simulink model "Kalman"  (R2019b)
settings: Solver=VariableStepAuto  StartTime=0.0  StopTime=20  RelTol=1e-3
values from neighbouring files (symbols this model uses):
  A = [0.01   -0.4940 ; 0.1129 -0.3832]    [Initialization.m]
  B = [0.5919 ; 0.5191]    [Initialization.m]
  C = [1 0]    [Initialization.m]
  mn = 0.07    [Initialization.m]
  pn = 0.09    [Initialization.m]
  Ts = -1    [Initialization.m]
undefined symbols (not defined in the file or in its folder): Continuous, sigbuilder_block, Time
libraries: ctrlSharedLib x1
settings Model: Creator=Devan  LastModifiedBy=Devan

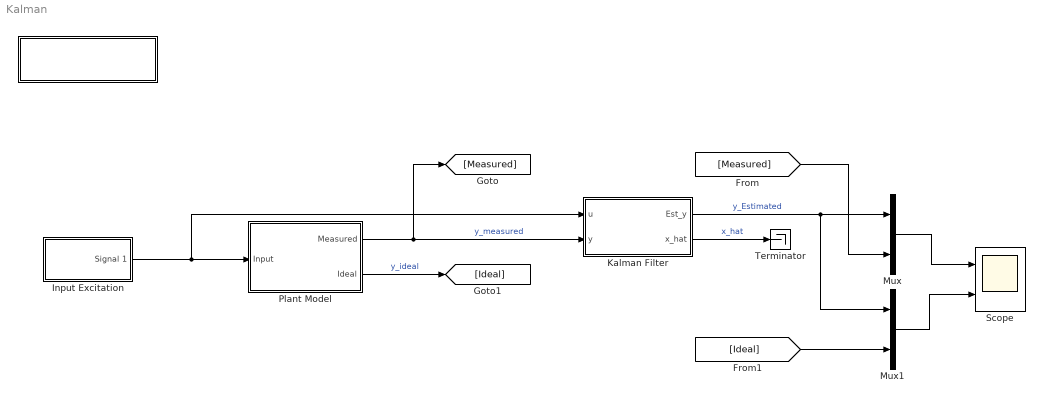
== system Kalman ==
  " " : Subsystem  LoadFcn=run('Initialization.m')  InitFcn=run('Initialization.m')
      settings: OpenFcn=run('Initialization.m')
      mask DialogControl Control3 Prompt: Click to Initialize System
      mask Display: disp('Click to Initialize System')
  Input Excitation : Subsystem  Tag=STV Subsys  LoadFcn=sigbuilder_block('load');  StartFcn=sigbuilder_block('start');  StopFcn=sigbuilder_block('stop');  ClipboardFcn=sigbuilder_block('clipboard');  mask(Sigbuilder block){tuvar=[0:10]}
      mask help: Simulink:masks:SigbuilderBlock_MD
      mask init:
      | if ~strcmp(get_param(bdroot(gcbh),'SimulationStatus'),'stopped') tuvar = sigbuilder_block('maskInit'); end
      settings: CopyFcn=sigbuilder_block('copy');  DeleteFcn=sigbuilder_block('delete');  ModelCloseFcn=sigbuilder_block('modelClose');  PreSaveFcn=sigbuilder_block('preSave');  PauseFcn=sigbuilder_block('pause');  ContinueFcn=sigbuilder_block('continue');  NameChangeFcn=sigbuilder_block('namechange');  OpenFcn=sigbuilder_block('open',[211.5 97.5 550.5 362.5 ]);  CloseFcn=sigbuilder_block('close');
      mask Display: plot(0, 0, 100, 100,[2, 2, 32, 32, 2], [68, 8, 8, 68, 68],[32, 2], [38, 38], [32, 19, 2],[53, 60, 44], [32, 17, 17, 2],[16, 16, 31, 31]);txt = getActiveGroup(gcbh);text(2, 100, txt,'verticalAlignment', 'top');
  Kalman Filter : Subsystem
      mask Display: disp('Kalman Filter')
  Mux : Mux  Inputs=2
  Mux1 : Mux  Inputs=2
  Plant Model : Subsystem
      mask Display: disp('Plant')
  Scope : Scope  NumInputPorts=2
  Terminator : Terminator
  wires:
  Input Excitation/1(Signal 1) -> Kalman Filter/1(u), Plant Model/1(Input)
  Mux/1 -> Scope/1
  Plant Model/1(Measured) -> [Measured], Kalman Filter/2(y)  "y_measured"
  Plant Model/2(Ideal) -> [Ideal]  "y_ideal"
  Kalman Filter/2(x_hat) -> Terminator/1  "x_hat"
  Kalman Filter/1(Est_y) -> Mux1/1, Mux/1  "y_Estimated"
  [Measured] -> Mux/2
  Mux1/1 -> Scope/2
  [Ideal] -> Mux1/2

== system Kalman/  ==

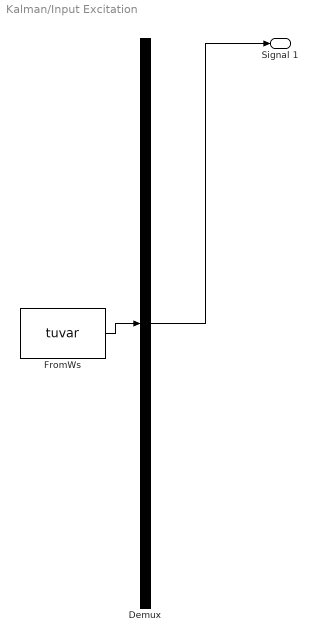
== system Kalman/Input Excitation ==
  Demux : Demux  Tag=STV Demux  Outputs=1
  FromWs : FromWorkspace  Tag=STV FromWs  VariableName=tuvar  SampleTime=0
      SigBuilderData=|
      | common.afterFinalStr = 'Extrapolate'
      | common.sampleTime = 0
      | dataSet.timeRange = [0 10]
      | dataSet.name = 'Group 1'
      | sbobj.Groups.Name = 'Group 1'
      | sbobj.Groups.Signals.Name = 'Signal 1'
      | sbobj.Groups.Signals.XData = [0 4 4 6 10]
      | sbobj.Groups.Signals.YData = [0 0 1 1 1]
  Signal 1 : Outport  Tag=STV Outport
  wires:
  Demux/1 -> Signal 1/1
  FromWs/1 -> Demux/1

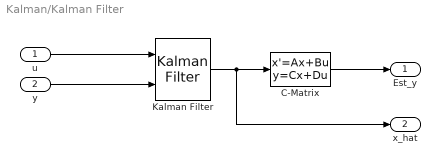
== system Kalman/Kalman Filter ==
  u : Inport
  y : Inport  Port=2
  C-Matrix : StateSpace  A=zeros(size(A))  B=zeros(size(A))  C=zeros(size(C))  D=C  InitialCondition=0
  Kalman Filter : ctrlSharedLib/Kalman Filter  TimeDomain=Continuous-Time  UseCurrentEstimator=on  ModelSource=Individual A, B, C, D matrices  ModelSourceVariable=ss(A,B,C,0)  A=A  B=B  C=C  D=0  NumberOfStates=1  NumberOfInputs=1  NumberOfOutputs=1  InitialEstimateSource=Dialog  X0=[0;0]  P0=10  UseK=off  UseGH=off  NumberOfProcessNoiseInputs=1  G=1  TimeInvariantG=on  H=0  TimeInvariantH=on  Q=pn  TimeInvariantQ=on  R=mn  TimeInvariantR=on  N=0  TimeInvariantN=on  AddInputPort=on  AddEnablePort=off  OutputEstimatedY=off  OutputP=off  Ts=-1
      settings: SourceProductBaseCode=CT
  Est_y : Outport
  x_hat : Outport  Port=2
  wires:
  y/1 -> Kalman Filter/2
  Kalman Filter/1 -> x_hat/1, C-Matrix/1
  C-Matrix/1 -> Est_y/1
  u/1 -> Kalman Filter/1

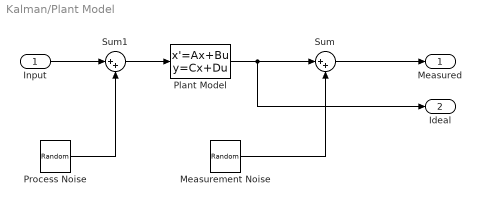
== system Kalman/Plant Model ==
  Input : Inport
  Measurement Noise : UniformRandomNumber  Minimum=-mn  Maximum=mn  SampleTime=Ts
  Plant Model : StateSpace  A=A  B=B  C=C  D=0  InitialCondition=[0;0]
  Process Noise : UniformRandomNumber  Minimum=-pn  Maximum=pn  SampleTime=Ts
  Sum : Sum  Inputs=|++
  Sum1 : Sum  Inputs=|++
  Measured : Outport
  Ideal : Outport  Port=2
  wires:
  Plant Model/1 -> Ideal/1, Sum/1
  Sum1/1 -> Plant Model/1
  Measurement Noise/1 -> Sum/2
  Sum/1 -> Measured/1
  Process Noise/1 -> Sum1/2
  Input/1 -> Sum1/1
